simulink model "ACCSampleSimulink"  (R2022a)
settings: Solver=ode1  StartTime=0.0  StopTime=inf  FixedStep=0.001  RelTol=1e-3
model workspace (MAT data in the model file):
  ParaDataStoreNum = Simulink.Parameter
  ParaDataStoreNum.DataType = 'int32'
  ParaDataStoreNum.Complexity = 'real'
  ParaDataStoreNum.Dimensions = [0 0]
undefined symbols (not defined in the file): azimuth_angle, DataStoreNumPara, elevation_angle, GroundTruth_Objects, heading, id, range_bbox, range_center, shape, time, type, velocity, width
(part 1 of 2)
Description:
  | 22222
settings Model: Creator=15751  LastModifiedBy=jwd
settings SolverCC: AlgebraicLoopSolver=TrustRegion
settings OptimizationCC: LifeSpan=inf
settings DebuggingCC: MultiTaskRateTransMsg=warning  UnconnectedInputMsg=warning  UnconnectedOutputMsg=warning  UnconnectedLineMsg=warning  SFExecutionAtInitializationDiag=none  SFMachineParentedDataDiag=warning  ArithmeticOperatorsInVariantConditions=warning
settings SFSimCC: CustomCodeUndefinedFunction=UseInterfaceOnly
settings CodeAppCC: StateflowObjectComments=on

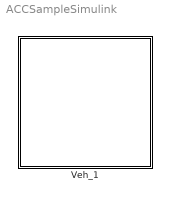
== system ACCSampleSimulink ==
  Veh_1 : Subsystem  Tag=PanoSim_System
      mask Display: image(imread('Sedan_2.jpg'));color('white');text(0,0,'Veh_1','HorizontalAlignment','left','verticalAlignment','bottom');color('red');text(0.1,0.1,'P','HorizontalAlignment','right','verticalAlignment','top');

== system ACCSampleSimulink/Veh_1 ==
  Algorithm : Subsystem
  AlgorithmControl : Subsystem
  ComplexVehicleModel : Subsystem
  Data Store Memory1 : DataStoreMemory  DataStoreName=DataStore_EGO_ALL  ReadBeforeWriteMsg=warning  WriteAfterWriteMsg=warning  WriteAfterReadMsg=warning  InitialValue=zeros(295,1)  ShowAdditionalParam=off  Dimensions=295
      settings: LockScale=on
  Data Store Memory2 : DataStoreMemory  DataStoreName=DataStore_COCKPIT_CONTROL  ReadBeforeWriteMsg=warning  WriteAfterWriteMsg=warning  WriteAfterReadMsg=warning  InitialValue=[0,0,0,0,0,0]  ShowAdditionalParam=off  Dimensions=6
      settings: LockScale=on
  Data Store Memory : DataStoreMemory  DataStoreName=DataStore_Ego_Control  ReadBeforeWriteMsg=warning  WriteAfterWriteMsg=warning  WriteAfterReadMsg=warning  InitialValue=[0,0,0,0,0,0]  ShowAdditionalParam=off  Dimensions=6
      settings: LockScale=on
  DriverModel : Subsystem  Tag=PanoSim_System
      mask Display: image(imread('driver.jpg'))
  GlobalVariable : Subsystem
  Sensors : Subsystem
  VehicleDataBus : Subsystem
  wires:
  Algorithm/3(LogDataOutput) -> VehicleDataBus/4(LogDataInput)
  Algorithm/2(GlobalVariableOutput) -> VehicleDataBus/2(GlobalVariable)
  Algorithm/1(ControlOutput) -> ComplexVehicleModel/1(Control)
  AlgorithmControl/1(AlgorithmControlOut) -> Algorithm/5(AlgorithmControlInput)
  GlobalVariable/1(Value) -> Algorithm/4(GlobalVariableInput)
  Sensors/1(SensorsOut) -> Algorithm/3(SensorsInput)
  DriverModel/1(DriverOut) -> Algorithm/2(ControlInput)
  [VehicleDynOut] -> Algorithm/1(VehDynInput)
  ComplexVehicleModel/1(Vehicle_Out) -> [VehicleDynOut], VehicleDataBus/1(VehicleDynOut)
  GlobalVariable/2(Original) -> VehicleDataBus/3(GlobalVariableOriginal)
  [VehicleDynOut] -> DriverModel/1(In1)

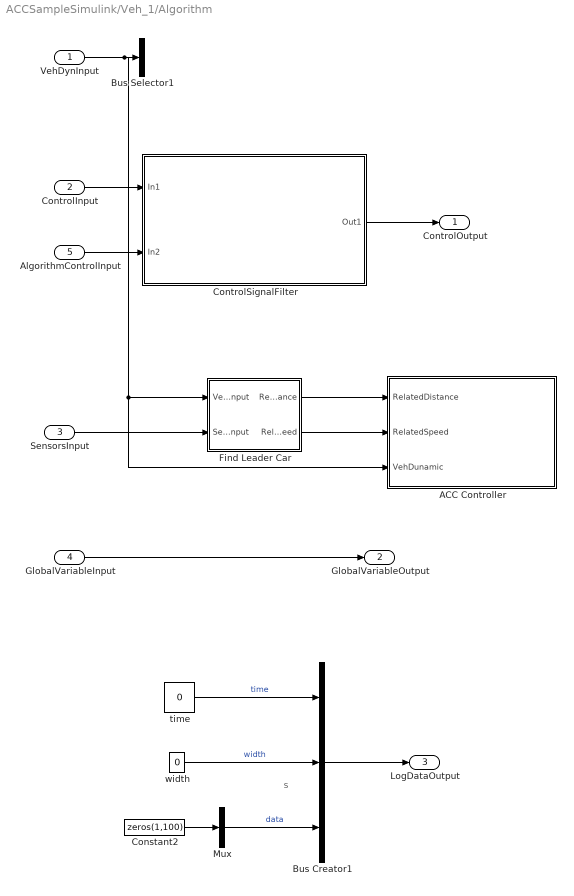
== system ACCSampleSimulink/Veh_1/Algorithm ==
  note: s
  VehDynInput : Inport
  ControlInput : Inport  Port=2
  SensorsInput : Inport  Port=3
  GlobalVariableInput : Inport  Port=4
  AlgorithmControlInput : Inport  Port=5
  " Find Leader Car" : Subsystem
  ACC Controller : Subsystem
  Bus Creator1 : BusCreator  Inputs=3
  Bus Selector1 : BusSelector  OutputSignals=ego
  Constant2 : Constant  Value=zeros(1,100)
  ControlSignalFilter : Subsystem
  Mux : Mux  Inputs=[100,]
  time : Constant  Value=0
  width : Constant  Value=0
  ControlOutput : Outport  VectorParamsAs1DForOutWhenUnconnected=off
  GlobalVariableOutput : Outport  Port=2  VectorParamsAs1DForOutWhenUnconnected=off
  LogDataOutput : Outport  Port=3  VectorParamsAs1DForOutWhenUnconnected=off
  wires:
  VehDynInput/1 -> ACC Controller/3(VehDunamic), " Find Leader Car"/1(VehDynInput), Bus Selector1/1
  ControlInput/1 -> ControlSignalFilter/1(In1)
  ControlSignalFilter/1(Out1) -> ControlOutput/1
  GlobalVariableInput/1 -> GlobalVariableOutput/1
  time/1 -> Bus Creator1/1  "time"
  Bus Creator1/1 -> LogDataOutput/1
  Constant2/1 -> Mux/1
  Mux/1 -> Bus Creator1/3  "data"
  width/1 -> Bus Creator1/2  "width"
  AlgorithmControlInput/1 -> ControlSignalFilter/2(In2)
  SensorsInput/1 -> " Find Leader Car"/2(SensorsInput)
  " Find Leader Car"/1(RelatedDistance) -> ACC Controller/1(RelatedDistance)
  " Find Leader Car"/2(RelatedSpeed) -> ACC Controller/2(RelatedSpeed)

== system ACCSampleSimulink/Veh_1/AlgorithmControl ==
  Bus{,2..5} (5 alike) : BusCreator  Inputs=3
  Bus1 : BusCreator  Inputs=5
  brake : S-Function  FunctionName=BusReader  Parameters='ego_control.brake','time@i,valid@b,brake@d','0.001','0.0'  SFunctionDeploymentMode=off  EnableBusSupport=off
  gear : S-Function  FunctionName=BusReader  Parameters='ego_control.gear','time@i,valid@b,gear@i','0.001','0.0'  SFunctionDeploymentMode=off  EnableBusSupport=off
  mode : S-Function  FunctionName=BusReader  Parameters='ego_control.mode','time@i,valid@b,mode@i','0.001','0.0'  SFunctionDeploymentMode=off  EnableBusSupport=off
  steer : S-Function  FunctionName=BusReader  Parameters='ego_control.steer','time@i,valid@b,steer@d','0.001','0.0'  SFunctionDeploymentMode=off  EnableBusSupport=off
  throttle : S-Function  FunctionName=BusReader  Parameters='ego_control.throttle','time@i,valid@b,throttle@d','0.001','0.0'  SFunctionDeploymentMode=off  EnableBusSupport=off
  AlgorithmControlOut : Outport  VectorParamsAs1DForOutWhenUnconnected=off
  wires:
  Bus1/1 -> AlgorithmControlOut/1
  Bus5/1 -> Bus1/1  "throttle"
  Bus4/1 -> Bus1/5  "gear"
  Bus3/1 -> Bus1/4  "mode"
  Bus2/1 -> Bus1/3  "steer"
  Bus/1 -> Bus1/2  "brake"
  gear/3 -> Bus4/3  "value"
  gear/2 -> Bus4/2  "valid"
  gear/1 -> Bus4/1  "time"
  mode/3 -> Bus3/3  "value"
  mode/2 -> Bus3/2  "valid"
  mode/1 -> Bus3/1  "time"
  steer/1 -> Bus2/1  "time"
  brake/1 -> Bus/1  "time"
  throttle/1 -> Bus5/1  "time"
  throttle/3 -> Bus5/3  "value"
  brake/3 -> Bus/3  "value"
  steer/3 -> Bus2/3  "value"
  throttle/2 -> Bus5/2  "valid"
  brake/2 -> Bus/2  "valid"
  steer/2 -> Bus2/2  "valid"

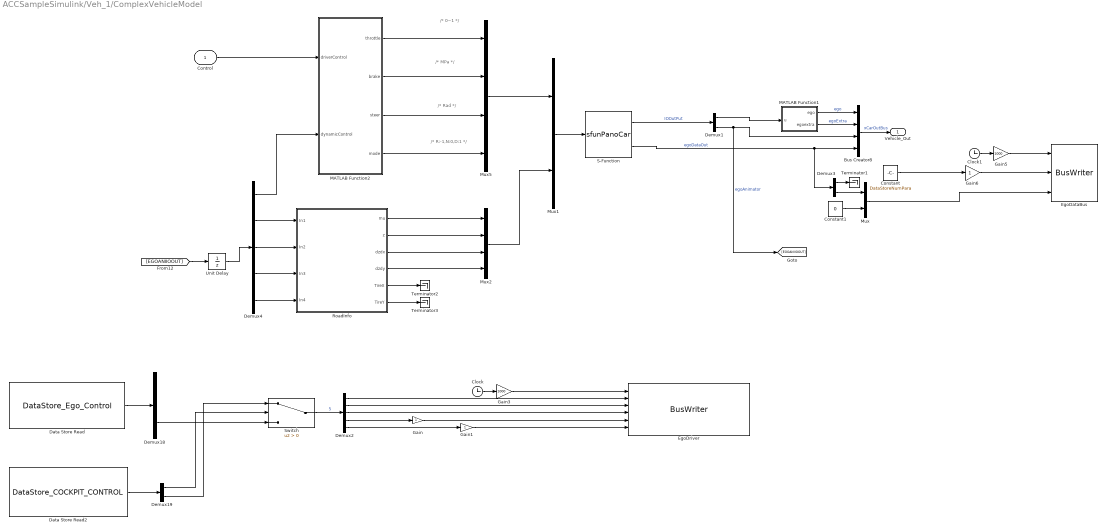
== system ACCSampleSimulink/Veh_1/ComplexVehicleModel ==
  note: /* MPa */
  note: /* 0~1 */
  note: /* R:-1,N:0,D:1 */
  note: /* Rad */
  Control : Inport
  Bus Creator8 : BusCreator  Inputs=4
  Clock : Clock
  Clock1 : Clock
  Constant : Constant  Value=DataStoreNumPara  VectorParams1D=off  OutDataTypeStr=double
  Constant1 : Constant  Value=0
  Data Store Read : DataStoreRead  DataStoreName=DataStore_Ego_Control  IndexOptions=Index vector (dialog)  Indices=1  OutputSizes=1
  Data Store Read2 : DataStoreRead  DataStoreName=DataStore_COCKPIT_CONTROL  IndexOptions=Index vector (dialog)  Indices=1  OutputSizes=1
  Demux1 : Demux  Outputs=[19,57]
  Demux18 : Demux  Outputs=[1,5]
  Demux19 : Demux  Outputs=[1,5]
  Demux2 : Demux  Outputs=5
  Demux3 : Demux  Outputs=[1,499]
  Demux4 : Demux  Outputs=[5,13,13,13,13]
  EgoDataBus : S-Function  FunctionName=BusWriter  Parameters='ego_data','time@i,500@[,data@d','0.01','0.0'  SFunctionDeploymentMode=off  EnableBusSupport=off
  EgoDriver : S-Function  FunctionName=BusWriter  Parameters='ego_driver','time@i,throttle@d,brake@d,steer@d,mode@i,gear@i','0.01','0.0'  SFunctionDeploymentMode=off  EnableBusSupport=off
  Gain : Gain  OutDataTypeStr=int32
  Gain1 : Gain  OutDataTypeStr=int32
  Gain3 : Gain  Gain=1000  OutDataTypeStr=Inherit: Inherit via back propagation  RndMeth=Nearest
  Gain5 : Gain  Gain=1000  OutDataTypeStr=Inherit: Inherit via back propagation  RndMeth=Nearest
  Gain6 : Gain  OutDataTypeStr=int32
  MATLAB Function1 : MATLAB Function  TreatAsAtomicUnit=on
  MATLAB Function2 : MATLAB Function  TreatAsAtomicUnit=on
  Mux : Mux  Inputs=[499,1]
  Mux1 : Mux  Inputs=[4,16]
  Mux2 : Mux
  Mux5 : Mux
  RoadInfo : Subsystem
  S-Function : S-Function  FunctionName=sfunPanoCar  SFunctionDeploymentMode=off  EnableBusSupport=off
  Switch : Switch  Criteria=u2 > Threshold  SaturateOnIntegerOverflow=off  InputSameDT=off
  Terminator1 : Terminator
  Terminator2 : Terminator
  Terminator3 : Terminator
  Unit Delay : UnitDelay  SampleTime=-1  HasFrameUpgradeWarning=on
  Vehicle_Out : Outport
  wires:
  MATLAB Function2/4(mode) -> Mux5/4
  MATLAB Function2/3(steer) -> Mux5/3
  MATLAB Function2/2(brake) -> Mux5/2
  MATLAB Function2/1(throttle) -> Mux5/1
  Demux4/4 -> RoadInfo/3(In3)
  Demux4/1 -> MATLAB Function2/2(dynamicControl)
  Demux4/2 -> RoadInfo/1(In1)
  Demux4/5 -> RoadInfo/4(In4)
  Unit Delay/1 -> Demux4/1
  Demux4/3 -> RoadInfo/2(In2)
  Mux/1 -> EgoDataBus/3
  Constant1/1 -> Mux/2
  Demux3/2 -> Mux/1
  Demux3/1 -> Terminator1/1
  Constant/1 -> Gain6/1
  Gain5/1 -> EgoDataBus/1
  Clock1/1 -> Gain5/1
  Gain6/1 -> EgoDataBus/2
  Demux19/2 -> Switch/1
  Data Store Read2/1 -> Demux19/1
  Data Store Read/1 -> Demux18/1
  Demux19/1 -> Switch/2
  Demux18/2 -> Switch/3
  Switch/1 -> Demux2/1  "5"
  Demux1/2 -> Bus Creator8/3, [EGOANIIOOUT]  "egoAnimator"
  MATLAB Function1/1(ego) -> Bus Creator8/1  "ego"
  Demux1/1 -> MATLAB Function1/1(u)
  MATLAB Function1/2(egoextra) -> Bus Creator8/2  "egoExtra"
  RoadInfo/6(TireY) -> Terminator3/1
  RoadInfo/5(TireX) -> Terminator2/1
  S-Function/2 -> Bus Creator8/4, Demux3/1  "egoDataOut"
  Gain1/1 -> EgoDriver/6
  Gain/1 -> EgoDriver/5
  Demux2/4 -> Gain/1
  Demux2/2 -> EgoDriver/3
  Control/1 -> MATLAB Function2/1(driverControl)
  Demux2/1 -> EgoDriver/2
  Demux2/3 -> EgoDriver/4
  Demux2/5 -> Gain1/1
  Gain3/1 -> EgoDriver/1
  Mux1/1 -> S-Function/1
  S-Function/1 -> Demux1/1  "IOOutPut"
  Bus Creator8/1 -> Vehicle_Out/1  "xCarOutBus"
  Mux5/1 -> Mux1/1
  Clock/1 -> Gain3/1
  Mux2/1 -> Mux1/2
  RoadInfo/3(dzdx) -> Mux2/3
  RoadInfo/1(mu) -> Mux2/1
  RoadInfo/2(z) -> Mux2/2
  RoadInfo/4(dzdy) -> Mux2/4
  [EGOANIIOOUT] -> Unit Delay/1

== system ACCSampleSimulink/Veh_1/DriverModel ==
  In1 : Inport
  DriverFilter : Subsystem
  DriverOut : Outport  VectorParamsAs1DForOutWhenUnconnected=off
  wires:
  DriverFilter/1(DriverOut) -> DriverOut/1

== system ACCSampleSimulink/Veh_1/GlobalVariable ==
  Bus : BusCreator  Inputs=2
  Variable : Subsystem
  Value : Outport  VectorParamsAs1DForOutWhenUnconnected=off
  Original : Outport  Port=2  VectorParamsAs1DForOutWhenUnconnected=off
  wires:
  Bus/1 -> Original/1
  Variable/2(Out2) -> Bus/2  "Time"
  Variable/1(Out1) -> Value/1, Bus/1  "Value"

== system ACCSampleSimulink/Veh_1/Sensors ==
  GroundTruth_Objects.0 : Subsystem
  SensorsBusCreator : BusCreator  Inputs=GroundTruth_Objects.0,
  sensor_template : Subsystem  Commented=on
  SensorsOut : Outport  VectorParamsAs1DForOutWhenUnconnected=off
  wires:
  SensorsBusCreator/1 -> SensorsOut/1
  GroundTruth_Objects.0/1(SensorOut) -> SensorsBusCreator/1  "GroundTruth_Objects.0"

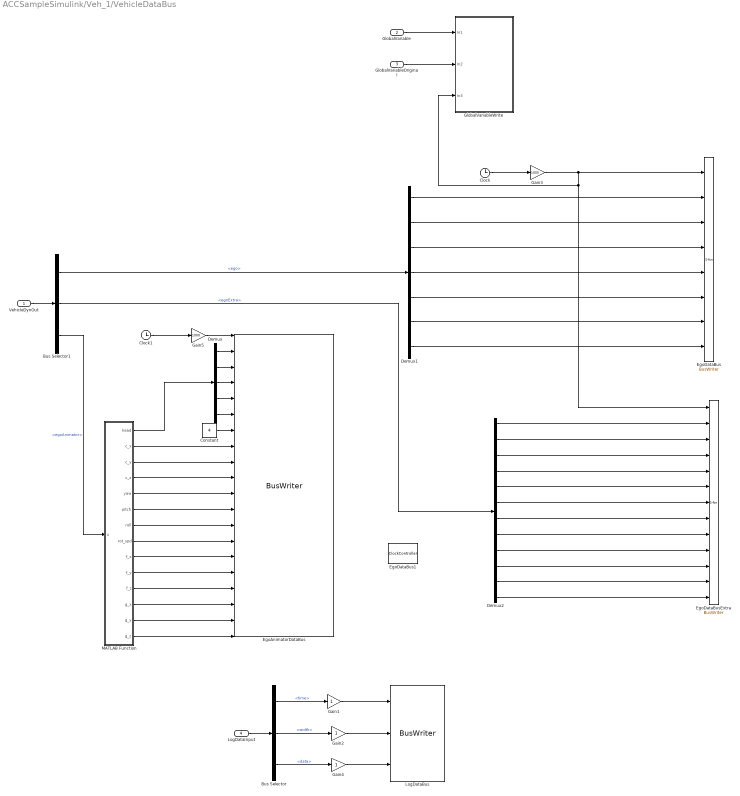
== system ACCSampleSimulink/Veh_1/VehicleDataBus ==
  VehicleDynOut : Inport
  GlobalVariable : Inport  Port=2
  GlobalVariableOriginal : Inport  Port=3
  LogDataInput : Inport  Port=4
  Bus Selector : BusSelector  OutputSignals=time,width,data
  Bus Selector1 : BusSelector  OutputSignals=ego,egoExtra,egoAnimator
  Clock : Clock
  Clock1 : Clock
  Constant : Constant  Value=4  OutDataTypeStr=int32
  Demux : Demux  Outputs=5
  Demux1 : Demux  Outputs=7
  Demux2 : Demux  Outputs=12
  EgoAnimatorDataBus : S-Function  FunctionName=BusWriter  Parameters='ego_animator','time@i,rot_spd@d,trans_gear@d,throttle@d,master@d,str@d,4@[,center_x@d,center_y@d,center_z@d,yaw@d,pitch@d,roll@d,rotation_spd@d,force_tire_x@d,force_tire_y@d,force_tire_z@d,gnd_x@d,gnd_y@d,gnd_z@d','0.01','0.0'  SFunctionDeploymentMode=off  EnableBusSupport=off
  EgoDataBus : S-Function  FunctionName=BusWriter  Parameters='ego','time@i,x@d,y@d,z@d,yaw@d,pitch@d,roll@d,speed@d','0.01','0.0'  SFunctionDeploymentMode=off  EnableBusSupport=off
  EgoDataBus1 : S-Function  FunctionName=ClockController  Parameters='step','0.01','0.0'  SFunctionDeploymentMode=off  EnableBusSupport=off
  EgoDataBusExtra : S-Function  FunctionName=BusWriter  Parameters='ego_extra','time@i,VX@d,VY@d,VZ@d,AVx@d,AVy@d,AVz@d,Ax@d,Ay@d,Az@d,AAx@d,AAy@d,AAz@d','0.01','0.0'  SFunctionDeploymentMode=off  EnableBusSupport=off
  Gain1 : Gain  OutDataTypeStr=int32  RndMeth=Nearest
  Gain2 : Gain  OutDataTypeStr=int32  RndMeth=Nearest
  Gain3 : Gain  Gain=1000  OutDataTypeStr=Inherit: Inherit via back propagation  RndMeth=Nearest
  Gain4 : Gain  OutDataTypeStr=double  RndMeth=Nearest
  Gain5 : Gain  Gain=1000  OutDataTypeStr=Inherit: Inherit via back propagation  RndMeth=Nearest
  GlobalVariableWrite : Subsystem
  LogDataBus : S-Function  FunctionName=BusWriter  Parameters='data','time@i,100@[,data@d','0.01','0.0'  SFunctionDeploymentMode=off  EnableBusSupport=off
  MATLAB Function : MATLAB Function  TreatAsAtomicUnit=on
  wires:
  Demux/5 -> EgoAnimatorDataBus/6
  MATLAB Function/14(g_z) -> EgoAnimatorDataBus/20
  MATLAB Function/13(g_y) -> EgoAnimatorDataBus/19
  MATLAB Function/12(g_x) -> EgoAnimatorDataBus/18
  MATLAB Function/11(f_z) -> EgoAnimatorDataBus/17
  MATLAB Function/10(f_y) -> EgoAnimatorDataBus/16
  MATLAB Function/9(f_x) -> EgoAnimatorDataBus/15
  MATLAB Function/8(rot_spd) -> EgoAnimatorDataBus/14
  MATLAB Function/7(roll) -> EgoAnimatorDataBus/13
  MATLAB Function/6(pitch) -> EgoAnimatorDataBus/12
  MATLAB Function/5(yaw) -> EgoAnimatorDataBus/11
  MATLAB Function/4(c_z) -> EgoAnimatorDataBus/10
  MATLAB Function/3(c_y) -> EgoAnimatorDataBus/9
  MATLAB Function/2(c_x) -> EgoAnimatorDataBus/8
  Constant/1 -> EgoAnimatorDataBus/7
  Demux/4 -> EgoAnimatorDataBus/5
  Demux/3 -> EgoAnimatorDataBus/4
  Demux/2 -> EgoAnimatorDataBus/3
  Demux/1 -> EgoAnimatorDataBus/2
  MATLAB Function/1(head) -> Demux/1
  Gain5/1 -> EgoAnimatorDataBus/1
  Clock1/1 -> Gain5/1
  Bus Selector1/3 -> MATLAB Function/1(u)  "<egoAnimator>"
  Bus Selector1/2 -> Demux2/1  "<egoExtra>"
  Bus Selector1/1 -> Demux1/1  "<ego>"
  Gain2/1 -> LogDataBus/2
  Bus Selector/2 -> Gain2/1  "<width>"
  Gain4/1 -> LogDataBus/3
  Bus Selector/1 -> Gain1/1  "<time>"
  Bus Selector/3 -> Gain4/1  "<data>"
  Gain1/1 -> LogDataBus/1
  LogDataInput/1 -> Bus Selector/1
  GlobalVariableOriginal/1 -> GlobalVariableWrite/2(In2)
  Gain3/1 -> EgoDataBus/1, EgoDataBusExtra/1, GlobalVariableWrite/3(In3)
  GlobalVariable/1 -> GlobalVariableWrite/1(In1)
  Demux2/12 -> EgoDataBusExtra/13
  Demux2/11 -> EgoDataBusExtra/12
  Demux2/10 -> EgoDataBusExtra/11
  Demux2/9 -> EgoDataBusExtra/10
  Demux2/8 -> EgoDataBusExtra/9
  Demux2/7 -> EgoDataBusExtra/8
  Demux2/6 -> EgoDataBusExtra/7
  Demux2/5 -> EgoDataBusExtra/6
  Demux2/4 -> EgoDataBusExtra/5
  Demux2/3 -> EgoDataBusExtra/4
  Demux2/2 -> EgoDataBusExtra/3
  Demux2/1 -> EgoDataBusExtra/2
  VehicleDynOut/1 -> Bus Selector1/1
  Clock/1 -> Gain3/1
  Demux1/1 -> EgoDataBus/2
  Demux1/2 -> EgoDataBus/3
  Demux1/3 -> EgoDataBus/4
  Demux1/4 -> EgoDataBus/5
  Demux1/5 -> EgoDataBus/6
  Demux1/6 -> EgoDataBus/7
  Demux1/7 -> EgoDataBus/8

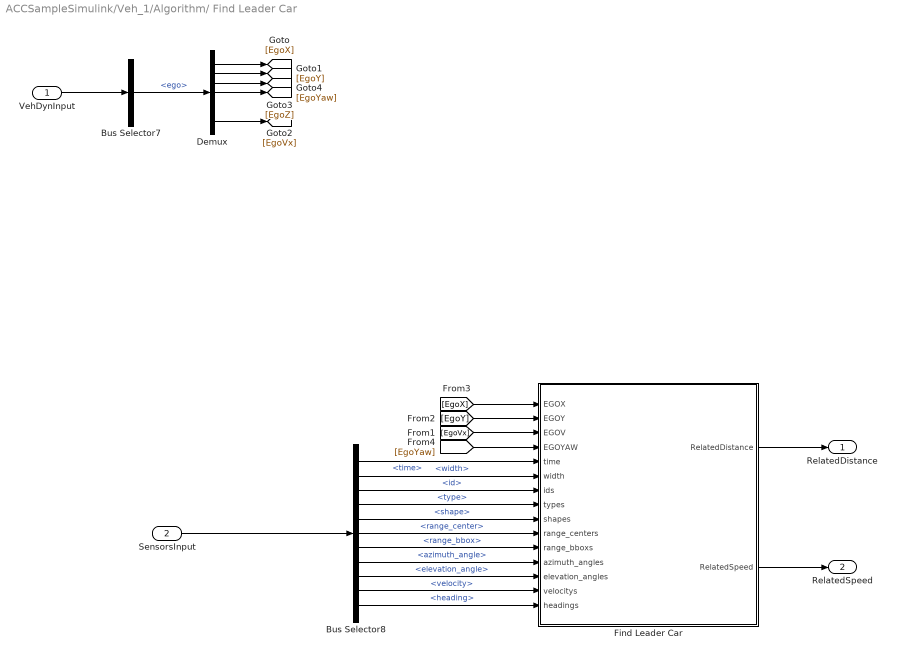
== system ACCSampleSimulink/Veh_1/Algorithm/ Find Leader Car ==
  VehDynInput : Inport
  SensorsInput : Inport  Port=2
  Bus Selector7 : BusSelector  OutputSignals=ego
  Bus Selector8 : BusSelector  OutputSignals=GroundTruth_Objects:0.time,GroundTruth_Objects:0.width,GroundTruth_Objects:0.id,GroundTruth_Objects:0.type,GroundTruth_Objects:0.shape,GroundTruth_Objects:0.range_center,GroundTruth_Objects:0.range_bbox,GroundTruth_Objects:0.azimuth_angle,GroundTruth_Objects:0.elevation_angle,GroundTruth_Objects:0.velocity,GroundTruth_Objects:0.heading
  Demux : Demux  Outputs=[1,1,1,1,1,1,1]
  Find Leader Car : MATLAB Function  TreatAsAtomicUnit=on
  RelatedDistance : Outport
  RelatedSpeed : Outport  Port=2
  wires:
  Find Leader Car/1(RelatedDistance) -> RelatedDistance/1
  Find Leader Car/2(RelatedSpeed) -> RelatedSpeed/1
  Bus Selector8/2 -> Find Leader Car/6(width)  "<width>"
  Bus Selector8/8 -> Find Leader Car/12(azimuth_angles)  "<azimuth_angle>"
  [EgoY] -> Find Leader Car/2(EGOY)
  Bus Selector8/1 -> Find Leader Car/5(time)  "<time>"
  [EgoX] -> Find Leader Car/1(EGOX)
  Bus Selector8/5 -> Find Leader Car/9(shapes)  "<shape>"
  Bus Selector8/4 -> Find Leader Car/8(types)  "<type>"
  Bus Selector8/3 -> Find Leader Car/7(ids)  "<id>"
  Bus Selector8/11 -> Find Leader Car/15(headings)  "<heading>"
  [EgoVx] -> Find Leader Car/3(EGOV)
  Bus Selector8/7 -> Find Leader Car/11(range_bboxs)  "<range_bbox>"
  [EgoYaw] -> Find Leader Car/4(EGOYAW)
  Bus Selector8/9 -> Find Leader Car/13(elevation_angles)  "<elevation_angle>"
  SensorsInput/1 -> Bus Selector8/1
  Bus Selector8/6 -> Find Leader Car/10(range_centers)  "<range_center>"
  Bus Selector8/10 -> Find Leader Car/14(velocitys)  "<velocity>"
  Demux/3 -> [EgoZ]
  Demux/1 -> [EgoX]
  Demux/7 -> [EgoVx]
  VehDynInput/1 -> Bus Selector7/1
  Demux/2 -> [EgoY]
  Demux/4 -> [EgoYaw]
  Bus Selector7/1 -> Demux/1  "<ego>"

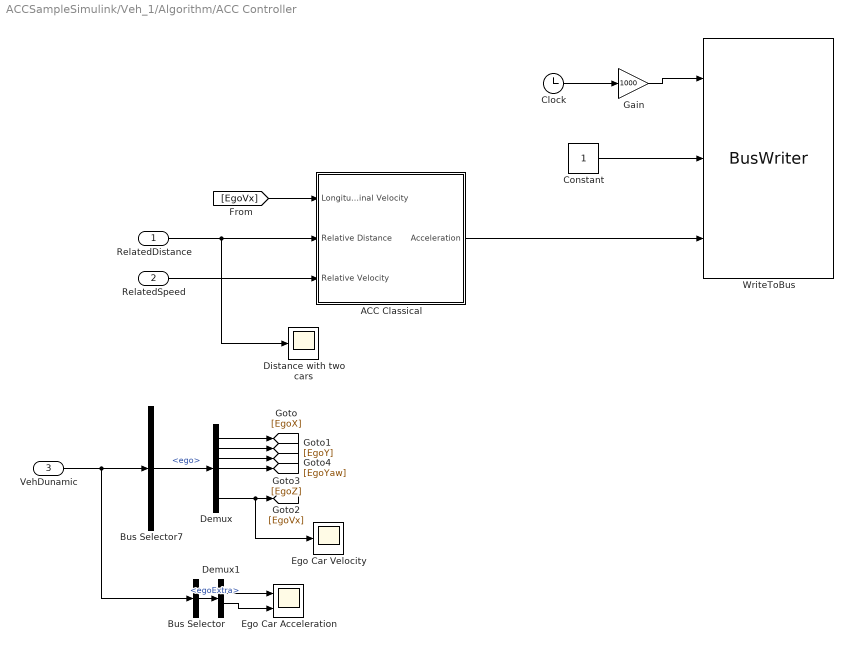
== system ACCSampleSimulink/Veh_1/Algorithm/ACC Controller ==
  RelatedDistance : Inport
  RelatedSpeed : Inport  Port=2
  VehDunamic : Inport  Port=3
  ACC Classical : Subsystem
  Bus Selector : BusSelector  OutputSignals=egoExtra
  Bus Selector7 : BusSelector  OutputSignals=ego
  Clock : Clock
  Constant : Constant  OutDataTypeStr=uint8
  Demux : Demux  Outputs=[1,1,1,1,1,1,1]
  Demux1 : Demux  Outputs=[6,1,1,4]
  Distance with two cars : Scope
  Ego Car Acceleration : Scope  NumInputPorts=2
  Ego Car Velocity : Scope
  Gain : Gain  Gain=1000  OutDataTypeStr=int32
  WriteToBus : S-Function  FunctionName=BusWriter  Parameters='xDriver_accel_input','time@i,valid@b,accel@d','0.01','0.0'  SFunctionDeploymentMode=off  EnableBusSupport=off
  wires:
  RelatedSpeed/1 -> ACC Classical/3("Relative Velocity ")
  RelatedDistance/1 -> Distance with two cars/1, ACC Classical/2(Relative Distance)
  Demux/1 -> [EgoX]
  Demux/4 -> [EgoYaw]
  Demux/2 -> [EgoY]
  VehDunamic/1 -> Bus Selector/1, Bus Selector7/1
  Demux/3 -> [EgoZ]
  [EgoVx] -> ACC Classical/1("Longitudinal Velocity ")
  Clock/1 -> Gain/1
  Gain/1 -> WriteToBus/1
  Constant/1 -> WriteToBus/2
  ACC Classical/1(" Acceleration") -> WriteToBus/3
  Bus Selector7/1 -> Demux/1  "<ego>"
  Demux1/3 -> Ego Car Acceleration/2
  Demux/7 -> Ego Car Velocity/1, [EgoVx]
  Bus Selector/1 -> Demux1/1  "<egoExtra>"
  Demux1/2 -> Ego Car Acceleration/1

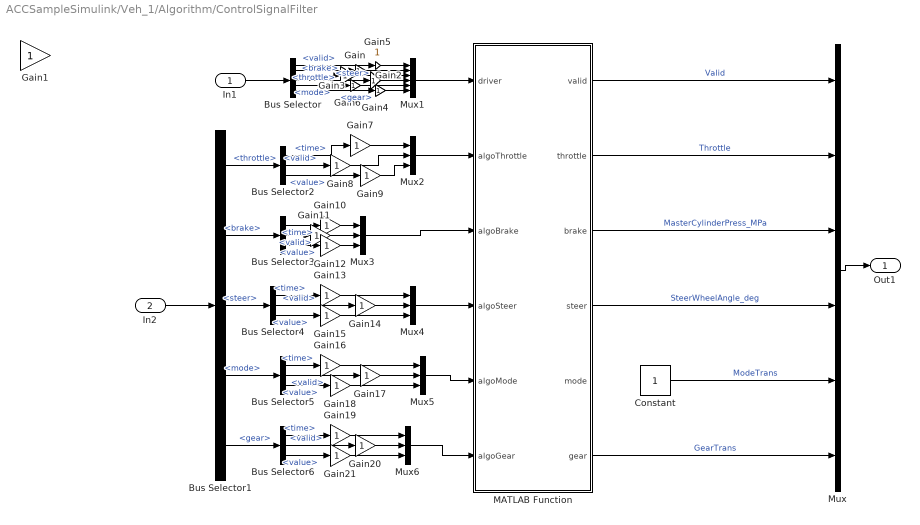
== system ACCSampleSimulink/Veh_1/Algorithm/ControlSignalFilter ==
  In1 : Inport
  In2 : Inport  Port=2
  Bus Selector : BusSelector  OutputSignals=valid,throttle,brake,steer,mode,gear
  Bus Selector1 : BusSelector  OutputSignals=throttle,brake,steer,mode,gear
  Bus Selector{2..6} (5 alike) : BusSelector  OutputSignals=time,valid,value
  Constant : Constant
  Gain{,2..21} (21 alike) : Gain  OutDataTypeStr=double
  Gain1 : Gain
  MATLAB Function : MATLAB Function  TreatAsAtomicUnit=on
  Mux : Mux  Inputs=6
  Mux1 : Mux  Inputs=6
  Mux{2..6} (5 alike) : Mux  Inputs=3
  Out1 : Outport  VectorParamsAs1DForOutWhenUnconnected=off
  wires:
  In1/1 -> Bus Selector/1
  Mux/1 -> Out1/1
  MATLAB Function/2(throttle) -> Mux/2  "Throttle"
  MATLAB Function/4(steer) -> Mux/4  "SteerWheelAngle_deg"
  MATLAB Function/1(valid) -> Mux/1  "Valid"
  Constant/1 -> Mux/5  "ModeTrans"
  MATLAB Function/6(gear) -> Mux/6  "GearTrans"
  In2/1 -> Bus Selector1/1
  Bus Selector1/1 -> Bus Selector2/1  "<throttle>"
  Bus Selector1/2 -> Bus Selector3/1  "<brake>"
  Bus Selector1/3 -> Bus Selector4/1  "<steer>"
  Bus Selector1/4 -> Bus Selector5/1  "<mode>"
  Bus Selector1/5 -> Bus Selector6/1  "<gear>"
  MATLAB Function/3(brake) -> Mux/3  "MasterCylinderPress_MPa"
  Bus Selector/1 -> Gain5/1  "<valid>"
  Bus Selector/2 -> Gain/1  "<throttle>"
  Bus Selector/3 -> Gain6/1  "<brake>"
  Bus Selector/4 -> Gain4/1  "<steer>"
  Bus Selector/5 -> Gain3/1  "<mode>"
  Bus Selector/6 -> Gain2/1  "<gear>"
  Mux1/1 -> MATLAB Function/1(driver)
  Bus Selector2/1 -> Gain7/1  "<time>"
  Bus Selector2/2 -> Gain8/1  "<valid>"
  Bus Selector2/3 -> Gain9/1  "<value>"
  Mux2/1 -> MATLAB Function/2(algoThrottle)
  Bus Selector3/1 -> Gain10/1  "<time>"
  Bus Selector3/2 -> Gain11/1  "<valid>"
  Bus Selector3/3 -> Gain12/1  "<value>"
  Mux3/1 -> MATLAB Function/3(algoBrake)
  Bus Selector4/1 -> Gain13/1  "<time>"
  Bus Selector4/2 -> Gain14/1  "<valid>"
  Bus Selector4/3 -> Gain15/1  "<value>"
  Mux4/1 -> MATLAB Function/4(algoSteer)
  Bus Selector5/1 -> Gain16/1  "<time>"
  Bus Selector5/2 -> Gain17/1  "<valid>"
  Bus Selector5/3 -> Gain18/1  "<value>"
  Mux5/1 -> MATLAB Function/5(algoMode)
  Bus Selector6/1 -> Gain19/1  "<time>"
  Bus Selector6/2 -> Gain20/1  "<valid>"
  Bus Selector6/3 -> Gain21/1  "<value>"
  Mux6/1 -> MATLAB Function/6(algoGear)
  Gain/1 -> Mux1/2
  Gain2/1 -> Mux1/6
  Gain3/1 -> Mux1/5
  Gain4/1 -> Mux1/4
  Gain5/1 -> Mux1/1
  Gain6/1 -> Mux1/3
  Gain7/1 -> Mux2/1
  Gain8/1 -> Mux2/2
  Gain9/1 -> Mux2/3
  Gain10/1 -> Mux3/1
  Gain11/1 -> Mux3/2
  Gain12/1 -> Mux3/3
  Gain13/1 -> Mux4/1
  Gain14/1 -> Mux4/2
  Gain15/1 -> Mux4/3
  Gain16/1 -> Mux5/1
  Gain17/1 -> Mux5/2
  Gain18/1 -> Mux5/3
  Gain19/1 -> Mux6/1
  Gain20/1 -> Mux6/2
  Gain21/1 -> Mux6/3

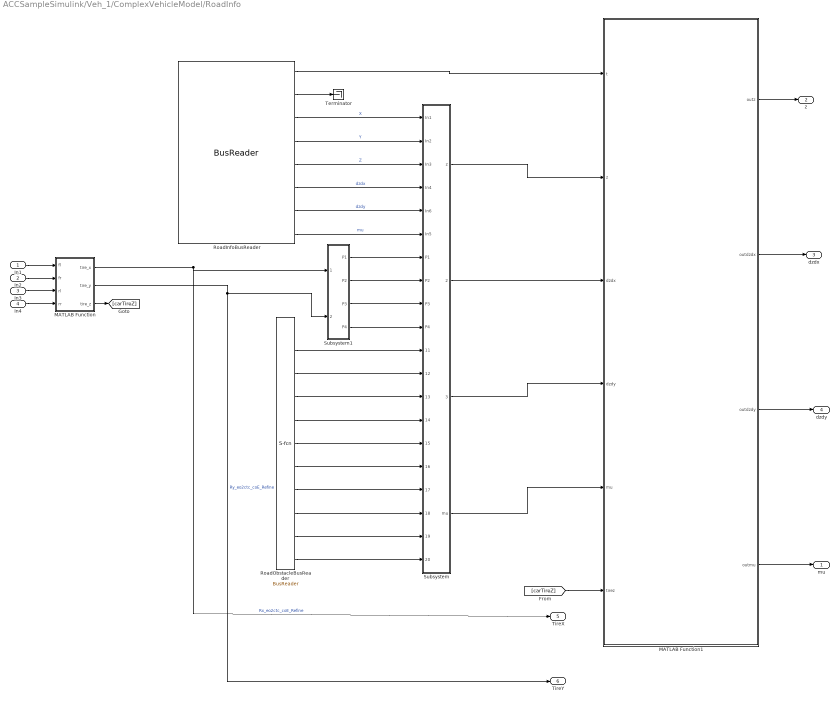
== system ACCSampleSimulink/Veh_1/ComplexVehicleModel/RoadInfo ==
  In1 : Inport
  In2 : Inport  Port=2
  In3 : Inport  Port=3
  In4 : Inport  Port=4
  MATLAB Function : MATLAB Function  TreatAsAtomicUnit=on
  MATLAB Function1 : MATLAB Function  TreatAsAtomicUnit=on
  RoadInfoBusReader : S-Function  FunctionName=BusReader  Parameters='road_info','time@i,16@[,x@d,y@d,z@d,dzdx@d,dzdy@d,mu@d','0.001','0.0'  SFunctionDeploymentMode=off  EnableBusSupport=off
  RoadObstacleBusReader : S-Function  FunctionName=BusReader  Parameters='road_obstacle','time@i,4@[,x1@d,y1@d,x2@d,y2@d,x3@d,y3@d,x4@d,y4@d,z@d','0.001','0.0'  SFunctionDeploymentMode=off  EnableBusSupport=off
  Subsystem : Subsystem
  Subsystem1 : Subsystem
  Terminator : Terminator
  mu : Outport  VectorParamsAs1DForOutWhenUnconnected=off
  z : Outport  Port=2  VectorParamsAs1DForOutWhenUnconnected=off
  dzdx : Outport  Port=3  VectorParamsAs1DForOutWhenUnconnected=off
  dzdy : Outport  Port=4  VectorParamsAs1DForOutWhenUnconnected=off
  TireX : Outport  Port=5  VectorParamsAs1DForOutWhenUnconnected=off
  TireY : Outport  Port=6  VectorParamsAs1DForOutWhenUnconnected=off
  wires:
  In1/1 -> MATLAB Function/1(fl)
  In2/1 -> MATLAB Function/2(fr)
  In3/1 -> MATLAB Function/3(rl)
  In4/1 -> MATLAB Function/4(rr)
  MATLAB Function1/4(outmu) -> mu/1
  MATLAB Function1/3(outdzdy) -> dzdy/1
  MATLAB Function1/2(outdzdx) -> dzdx/1
  MATLAB Function1/1(outz) -> z/1
  [carTireZ] -> MATLAB Function1/6(tirez)
  RoadInfoBusReader/1 -> MATLAB Function1/1(t)
  RoadInfoBusReader/2 -> Terminator/1
  MATLAB Function/3(tire_z) -> [carTireZ]
  RoadObstacleBusReader/11 -> Subsystem/20(In20)
  RoadObstacleBusReader/10 -> Subsystem/19(In19)
  RoadObstacleBusReader/9 -> Subsystem/18(In18)
  RoadObstacleBusReader/8 -> Subsystem/17(In17)
  RoadObstacleBusReader/7 -> Subsystem/16(In16)
  RoadObstacleBusReader/6 -> Subsystem/15(In15)
  RoadObstacleBusReader/5 -> Subsystem/14(In14)
  RoadObstacleBusReader/4 -> Subsystem/13(In13)
  RoadObstacleBusReader/3 -> Subsystem/12(In12)
  RoadObstacleBusReader/2 -> Subsystem/11(In11)
  RoadInfoBusReader/3 -> Subsystem/1(In1)  "X"
  RoadInfoBusReader/4 -> Subsystem/2(In2)  "Y"
  RoadInfoBusReader/5 -> Subsystem/3(In3)  "Z"
  RoadInfoBusReader/6 -> Subsystem/4(In4)  "dzdx"
  RoadInfoBusReader/7 -> Subsystem/5(In6)  "dzdy"
  RoadInfoBusReader/8 -> Subsystem/6(In5)  "mu"
  Subsystem/4(mu) -> MATLAB Function1/5(mu)
  Subsystem/3(dzdy) -> MATLAB Function1/4(dzdy)
  Subsystem/1(z) -> MATLAB Function1/2(z)
  Subsystem/2(dzdx) -> MATLAB Function1/3(dzdx)
  MATLAB Function/2(tire_y) -> Subsystem1/2(Ry_eo2ctc_coE_Refine), TireY/1  "Ry_eo2ctc_coE_Refine"
  MATLAB Function/1(tire_x) -> Subsystem1/1(Rx_eo2ctc_coE_Refine), TireX/1  "Rx_eo2ctc_coE_Refine"
  Subsystem1/1(P1) -> Subsystem/7(P1)
  Subsystem1/2(P2) -> Subsystem/8(P2)
  Subsystem1/3(P3) -> Subsystem/9(P3)
  Subsystem1/4(P4) -> Subsystem/10(P4)

== system ACCSampleSimulink/Veh_1/DriverModel/DriverFilter ==
  note: DriverBusCreator
  Bus Creator2 : BusCreator  Inputs=6
  Bus Selector : BusSelector  OutputSignals=valid,throttle,brake,steer,mode,gear
  Data Store Write : DataStoreWrite  DataStoreName=DataStore_Ego_Control  IndexOptions=Index vector (dialog)  Indices=1  OutputSizes=1
  EgoControlBus : S-Function  FunctionName=BusReader  Parameters='ego_control','time@i,valid@b,throttle@d,brake@d,steer@d,mode@i,gear@i','0.001','0.0'  SFunctionDeploymentMode=off  EnableBusSupport=off
  Gain : Gain  OutDataTypeStr=double
  Gain1 : Gain  OutDataTypeStr=double
  Gain2 : Gain  OutDataTypeStr=double
  Mux : Mux  Inputs=6
  DriverOut : Outport  VectorParamsAs1DForOutWhenUnconnected=off
  wires:
  Bus Selector/6 -> Gain1/1  "<gear>"
  Bus Selector/1 -> Gain2/1  "<valid>"
  Bus Creator2/1 -> DriverOut/1, Bus Selector/1
  Gain/1 -> Mux/5
  Bus Selector/2 -> Mux/2  "<throttle>"
  Bus Selector/5 -> Gain/1  "<mode>"
  Gain1/1 -> Mux/6
  Gain2/1 -> Mux/1
  Bus Selector/4 -> Mux/4  "<steer>"
  Mux/1 -> Data Store Write/1
  Bus Selector/3 -> Mux/3  "<brake>"
  EgoControlBus/4 -> Bus Creator2/3  "brake"
  EgoControlBus/5 -> Bus Creator2/4  "steer"
  EgoControlBus/3 -> Bus Creator2/2  "throttle"
  EgoControlBus/2 -> Bus Creator2/1  "valid"
  EgoControlBus/6 -> Bus Creator2/5  "mode"
  EgoControlBus/7 -> Bus Creator2/6  "gear"

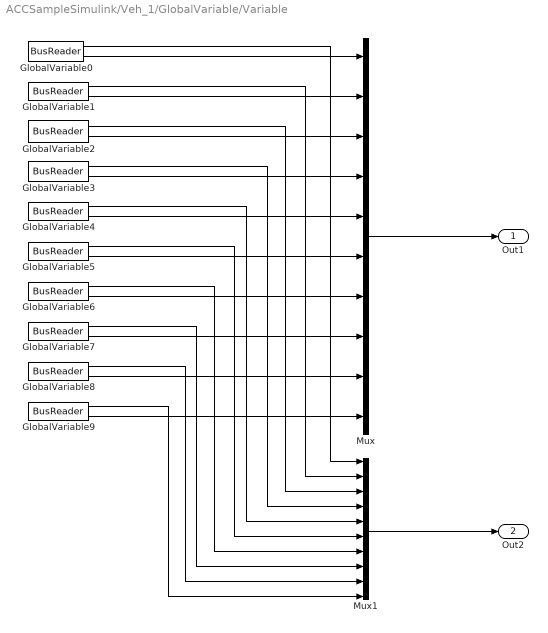
== system ACCSampleSimulink/Veh_1/GlobalVariable/Variable ==
  GlobalVariable0 : S-Function  FunctionName=BusReader  Parameters='global.0','time@i,variable@d','0.01','0.0'  SFunctionDeploymentMode=off  EnableBusSupport=off
  GlobalVariable1 : S-Function  FunctionName=BusReader  Parameters='global.1','time@i,variable@d','0.01','0.0'  SFunctionDeploymentMode=off  EnableBusSupport=off
  GlobalVariable2 : S-Function  FunctionName=BusReader  Parameters='global.2','time@i,variable@d','0.01','0.0'  SFunctionDeploymentMode=off  EnableBusSupport=off
  GlobalVariable3 : S-Function  FunctionName=BusReader  Parameters='global.3','time@i,variable@d','0.01','0.0'  SFunctionDeploymentMode=off  EnableBusSupport=off
  GlobalVariable4 : S-Function  FunctionName=BusReader  Parameters='global.4','time@i,variable@d','0.01','0.0'  SFunctionDeploymentMode=off  EnableBusSupport=off
  GlobalVariable5 : S-Function  FunctionName=BusReader  Parameters='global.5','time@i,variable@d','0.01','0.0'  SFunctionDeploymentMode=off  EnableBusSupport=off
  GlobalVariable6 : S-Function  FunctionName=BusReader  Parameters='global.6','time@i,variable@d','0.01','0.0'  SFunctionDeploymentMode=off  EnableBusSupport=off
  GlobalVariable7 : S-Function  FunctionName=BusReader  Parameters='global.7','time@i,variable@d','0.01','0.0'  SFunctionDeploymentMode=off  EnableBusSupport=off
  GlobalVariable8 : S-Function  FunctionName=BusReader  Parameters='global.8','time@i,variable@d','0.01','0.0'  SFunctionDeploymentMode=off  EnableBusSupport=off
  GlobalVariable9 : S-Function  FunctionName=BusReader  Parameters='global.9','time@i,variable@d','0.01','0.0'  SFunctionDeploymentMode=off  EnableBusSupport=off
  Mux : Mux  Inputs=10
  Mux1 : Mux  Inputs=10
  Out1 : Outport  VectorParamsAs1DForOutWhenUnconnected=off
  Out2 : Outport  Port=2  VectorParamsAs1DForOutWhenUnconnected=off
  wires:
  GlobalVariable9/1 -> Mux1/10
  GlobalVariable8/1 -> Mux1/9
  GlobalVariable7/1 -> Mux1/8
  GlobalVariable6/1 -> Mux1/7
  GlobalVariable5/1 -> Mux1/6
  GlobalVariable4/1 -> Mux1/5
  GlobalVariable3/1 -> Mux1/4
  GlobalVariable2/1 -> Mux1/3
  GlobalVariable1/1 -> Mux1/2
  GlobalVariable0/1 -> Mux1/1
  Mux1/1 -> Out2/1
  GlobalVariable9/2 -> Mux/10
  GlobalVariable8/2 -> Mux/9
  GlobalVariable7/2 -> Mux/8
  GlobalVariable6/2 -> Mux/7
  GlobalVariable5/2 -> Mux/6
  GlobalVariable4/2 -> Mux/5
  GlobalVariable3/2 -> Mux/4
  GlobalVariable2/2 -> Mux/3
  GlobalVariable1/2 -> Mux/2
  Mux/1 -> Out1/1
  GlobalVariable0/2 -> Mux/1

== system ACCSampleSimulink/Veh_1/Sensors/GroundTruth_Objects.0 ==
  BusCreator : BusCreator  Inputs=time,width,id,type,shape,range_center,range_bbox,azimuth_angle,elevation_angle,velocity,heading
  SensorBus : S-Function  FunctionName=BusReader  Parameters='GroundTruth_Objects.0','time@i,100@[,id@i,type@b,shape@i,range_center@f,range_bbox@f,azimuth_angle@f,elevation_angle@f,velocity@f,heading@f','0.01','0.0'  SFunctionDeploymentMode=off  EnableBusSupport=off
  SensorOut : Outport  VectorParamsAs1DForOutWhenUnconnected=off
  wires:
  SensorBus/11 -> BusCreator/11  "heading"
  SensorBus/10 -> BusCreator/10  "velocity"
  SensorBus/9 -> BusCreator/9  "elevation_angle"
  SensorBus/8 -> BusCreator/8  "azimuth_angle"
  SensorBus/7 -> BusCreator/7  "range_bbox"
  SensorBus/6 -> BusCreator/6  "range_center"
  SensorBus/5 -> BusCreator/5  "shape"
  SensorBus/4 -> BusCreator/4  "type"
  SensorBus/3 -> BusCreator/3  "id"
  SensorBus/2 -> BusCreator/2  "width"
  SensorBus/1 -> BusCreator/1  "time"
  BusCreator/1 -> SensorOut/1

== system ACCSampleSimulink/Veh_1/Sensors/sensor_template ==
  BusCreator : BusCreator  Inputs=8
  SensorBus : S-Function  FunctionName=BusReader  Parameters='mmwradar.0','time@i,64@[,angle@d,distance@d,speed@d,type@b,energy@d,id@i','0.1','0.0'  SFunctionDeploymentMode=off  EnableBusSupport=off
  SensorOut : Outport  VectorParamsAs1DForOutWhenUnconnected=off
  wires:
  BusCreator/1 -> SensorOut/1

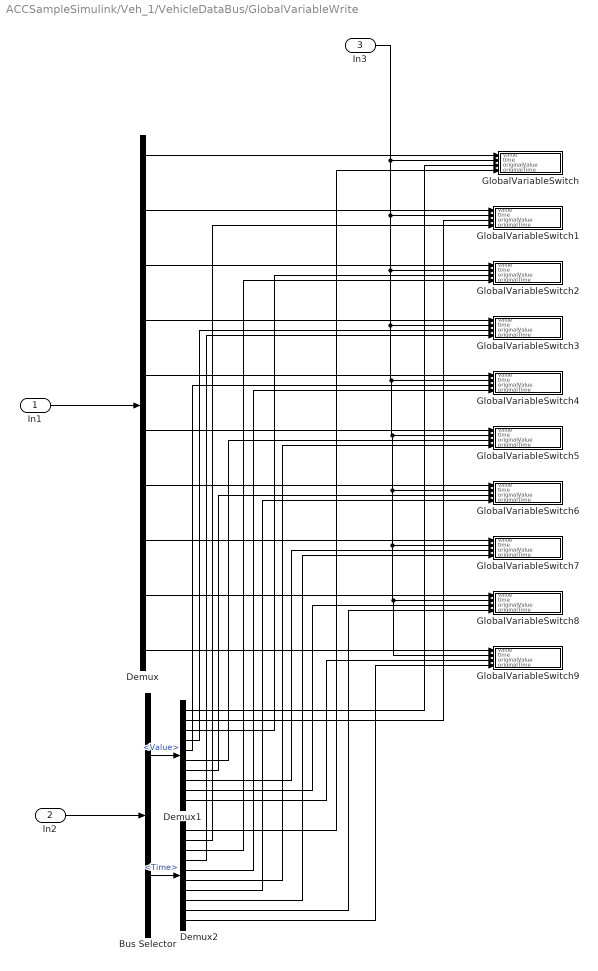
== system ACCSampleSimulink/Veh_1/VehicleDataBus/GlobalVariableWrite ==
  In1 : Inport
  In2 : Inport  Port=2
  In3 : Inport  Port=3
  Bus Selector : BusSelector  OutputSignals=Value,Time
  Demux : Demux  Outputs=10
  Demux1 : Demux  Outputs=10
  Demux2 : Demux  Outputs=10
  GlobalVariableSwitch : Subsystem
  GlobalVariableSwitch1 : Subsystem
  GlobalVariableSwitch2 : Subsystem
  GlobalVariableSwitch3 : Subsystem
  GlobalVariableSwitch4 : Subsystem
  GlobalVariableSwitch5 : Subsystem
  GlobalVariableSwitch6 : Subsystem
  GlobalVariableSwitch7 : Subsystem
  GlobalVariableSwitch8 : Subsystem
  GlobalVariableSwitch9 : Subsystem
  wires:
  Demux2/10 -> GlobalVariableSwitch9/4(originalTime)
  Demux1/10 -> GlobalVariableSwitch9/3(originalValue)
  Demux/10 -> GlobalVariableSwitch9/1(value)
  Demux2/9 -> GlobalVariableSwitch8/4(originalTime)
  Demux1/9 -> GlobalVariableSwitch8/3(originalValue)
  Demux/9 -> GlobalVariableSwitch8/1(value)
  Demux2/8 -> GlobalVariableSwitch7/4(originalTime)
  Demux1/8 -> GlobalVariableSwitch7/3(originalValue)
  Demux/8 -> GlobalVariableSwitch7/1(value)
  Demux2/7 -> GlobalVariableSwitch6/4(originalTime)
  Demux1/7 -> GlobalVariableSwitch6/3(originalValue)
  Demux/7 -> GlobalVariableSwitch6/1(value)
  Demux2/6 -> GlobalVariableSwitch5/4(originalTime)
  Demux1/6 -> GlobalVariableSwitch5/3(originalValue)
  Demux/6 -> GlobalVariableSwitch5/1(value)
  Demux2/5 -> GlobalVariableSwitch4/4(originalTime)
  Demux1/5 -> GlobalVariableSwitch4/3(originalValue)
  Demux/5 -> GlobalVariableSwitch4/1(value)
  Demux2/4 -> GlobalVariableSwitch3/4(originalTime)
  Demux1/4 -> GlobalVariableSwitch3/3(originalValue)
  Demux/4 -> GlobalVariableSwitch3/1(value)
  Demux2/3 -> GlobalVariableSwitch2/4(originalTime)
  Demux1/3 -> GlobalVariableSwitch2/3(originalValue)
  Demux/3 -> GlobalVariableSwitch2/1(value)
  Demux2/2 -> GlobalVariableSwitch1/4(originalTime)
  Demux1/2 -> GlobalVariableSwitch1/3(originalValue)
  Demux/2 -> GlobalVariableSwitch1/1(value)
  Demux2/1 -> GlobalVariableSwitch/4(originalTime)
  Demux1/1 -> GlobalVariableSwitch/3(originalValue)
  Demux/1 -> GlobalVariableSwitch/1(value)
  Bus Selector/2 -> Demux2/1  "<Time>"
  Bus Selector/1 -> Demux1/1  "<Value>"
  In2/1 -> Bus Selector/1
  In1/1 -> Demux/1
  In3/1 -> GlobalVariableSwitch/2(time), GlobalVariableSwitch1/2(time), GlobalVariableSwitch2/2(time), GlobalVariableSwitch3/2(time), GlobalVariableSwitch4/2(time), GlobalVariableSwitch5/2(time), GlobalVariableSwitch6/2(time), GlobalVariableSwitch7/2(time), GlobalVariableSwitch8/2(time), GlobalVariableSwitch9/2(time)

== system ACCSampleSimulink/Veh_1/Algorithm/ACC Controller/ACC Classical ==
  "Longitudinal Velocity " : Inport
  Relative Distance : Inport  Port=2
  "Relative Velocity " : Inport  Port=3
  ACC Classical : Subsystem  TreatAsAtomicUnit=on  VariantControl=controller_type == 1
      settings: RTWFileNameOpts=Use function name
  " Acceleration" : Outport  VectorParamsAs1DForOutWhenUnconnected=off
  wires:
  "Longitudinal Velocity "/1 -> ACC Classical/1(Longitudinal Velocity)
  Relative Distance/1 -> ACC Classical/2(Relative Distance)
  "Relative Velocity "/1 -> ACC Classical/3(Relative Velocity)
  ACC Classical/1(Acceleration) -> " Acceleration"/1

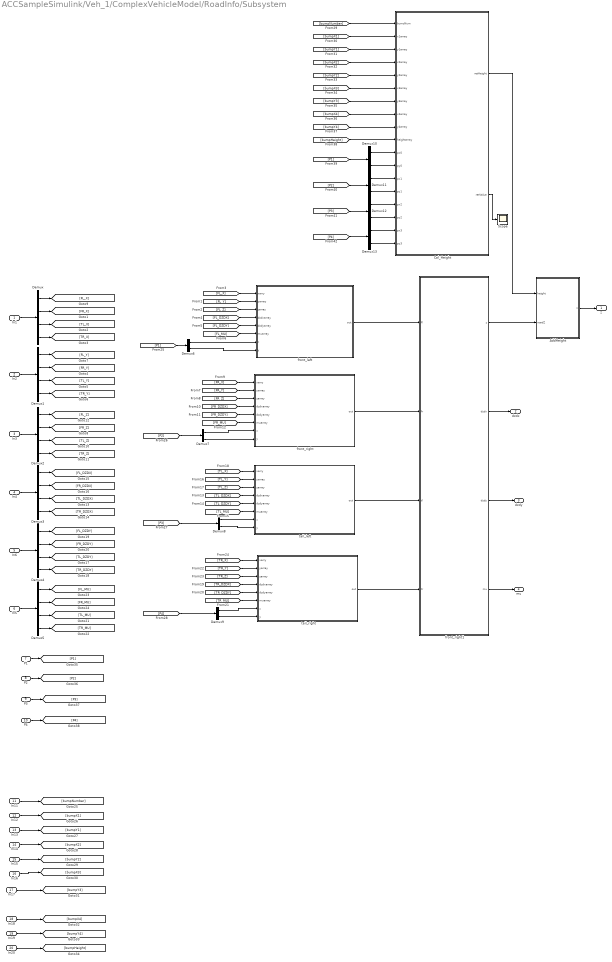
== system ACCSampleSimulink/Veh_1/ComplexVehicleModel/RoadInfo/Subsystem ==
  In1 : Inport
  In2 : Inport  Port=2
  In3 : Inport  Port=3
  In4 : Inport  Port=4
  In6 : Inport  Port=5
  In5 : Inport  Port=6
  P1 : Inport  Port=7
  P2 : Inport  Port=8
  P3 : Inport  Port=9
  P4 : Inport  Port=10
  In11 : Inport  Port=11
  In12 : Inport  Port=12
  In13 : Inport  Port=13
  In14 : Inport  Port=14
  In15 : Inport  Port=15
  In16 : Inport  Port=16
  In17 : Inport  Port=17
  In18 : Inport  Port=18
  In19 : Inport  Port=19
  In20 : Inport  Port=20
  AddHeight : MATLAB Function  TreatAsAtomicUnit=on
  Cal_Height : MATLAB Function  TreatAsAtomicUnit=on
  Demux{,1..5} (6 alike) : Demux
  Demux{6..13} (8 alike) : Demux  Outputs=2
  Scope : Scope
  front_left : MATLAB Function  TreatAsAtomicUnit=on
  front_right : MATLAB Function  TreatAsAtomicUnit=on
  front_right1 : MATLAB Function  TreatAsAtomicUnit=on
  tail_left : MATLAB Function  TreatAsAtomicUnit=on
  tail_right : MATLAB Function  TreatAsAtomicUnit=on
  z : Outport  VectorParamsAs1DForOutWhenUnconnected=off
  dzdx : Outport  Port=2  VectorParamsAs1DForOutWhenUnconnected=off
  dzdy : Outport  Port=3  VectorParamsAs1DForOutWhenUnconnected=off
  mu : Outport  Port=4  VectorParamsAs1DForOutWhenUnconnected=off
  wires:
  Cal_Height/2(retValue) -> Scope/1
  AddHeight/1(z) -> z/1
  Cal_Height/1(retHeight) -> AddHeight/1(height)
  [bumpY3] -> Cal_Height/7(y3array)
  Demux11/1 -> Cal_Height/13(px1)
  [bumpHeight] -> Cal_Height/10(heightarray)
  [bumpX1] -> Cal_Height/2(x1array)
  Demux11/2 -> Cal_Height/14(py1)
  [bumpY1] -> Cal_Height/3(y1array)
  [P2] -> Demux11/1
  Demux10/1 -> Cal_Height/11(px0)
  [bumpX3] -> Cal_Height/6(x3array)
  [P3] -> Demux12/1
  Demux10/2 -> Cal_Height/12(py0)
  [bumpNumber] -> Cal_Height/1(bumsNum)
  Demux12/1 -> Cal_Height/15(px2)
  [P4] -> Demux13/1
  Demux12/2 -> Cal_Height/16(py2)
  [bumpY4] -> Cal_Height/9(y4array)
  [bumpX4] -> Cal_Height/8(x4array)
  [P1] -> Demux10/1
  [bumpX2] -> Cal_Height/4(x2array)
  Demux13/1 -> Cal_Height/17(px3)
  Demux13/2 -> Cal_Height/18(py3)
  [bumpY2] -> Cal_Height/5(y2array)
  [P4] -> Demux9/1
  [P3] -> Demux8/1
  [P2] -> Demux7/1
  [P1] -> Demux6/1
  In20/1 -> [bumpHeight]
  In19/1 -> [bumpY4]
  In18/1 -> [bumpX4]
  In17/1 -> [bumpY3]
  In16/1 -> [bumpX3]
  In15/1 -> [bumpY2]
  In14/1 -> [bumpX2]
  In13/1 -> [bumpY1]
  In12/1 -> [bumpX1]
  In11/1 -> [bumpNumber]
  In1/1 -> Demux/1
  Demux/1 -> [FL_X]
  Demux/2 -> [FR_X]
  Demux/3 -> [TL_X]
  Demux/4 -> [TR_X]
  Demux1/1 -> [FL_Y]
  Demux1/3 -> [TL_Y]
  Demux1/4 -> [TR_Y]
  Demux1/2 -> [FR_Y]
  In2/1 -> Demux1/1
  In3/1 -> Demux2/1
  Demux2/4 -> [TR_Z]
  Demux2/3 -> [TL_Z]
  Demux2/2 -> [FR_Z]
  Demux2/1 -> [FL_Z]
  Demux3/4 -> [TR_DZDX]
  In4/1 -> Demux3/1
  Demux3/3 -> [TL_DZDX]
  Demux3/1 -> [FL_DZDX]
  Demux3/2 -> [FR_DZDX]
  Demux4/2 -> [FR_DZDY]
  Demux4/4 -> [TR_DZDY]
  Demux4/1 -> [FL_DZDY]
  Demux4/3 -> [TL_DZDY]
  In6/1 -> Demux4/1
  Demux5/3 -> [TL_MU]
  Demux5/4 -> [TR_MU]
  Demux5/2 -> [FR_MU]
  Demux5/1 -> [FL_MU]
  In5/1 -> Demux5/1
  [FL_X] -> front_left/1(xarry)
  [FL_Y] -> front_left/2(yarray)
  [FL_MU] -> front_left/6(muarray)
  [FL_DZDY] -> front_left/5(dzdyarray)
  [FL_DZDX] -> front_left/4(dzdxarray)
  [FL_Z] -> front_left/3(zarray)
  [FR_X] -> front_right/1(xarry)
  [FR_Y] -> front_right/2(yarray)
  [FR_Z] -> front_right/3(zarray)
  [FR_DZDX] -> front_right/4(dzdxarray)
  [FR_DZDY] -> front_right/5(dzdyarray)
  [FR_MU] -> front_right/6(muarray)
  [TL_X] -> tail_left/1(xarry)
  [TL_Y] -> tail_left/2(yarray)
  [TL_Z] -> tail_left/3(zarray)
  [TL_DZDX] -> tail_left/4(dzdxarray)
  [TL_DZDY] -> tail_left/5(dzdyarray)
  [TL_MU] -> tail_left/6(muarray)
  [TR_X] -> tail_right/1(xarry)
  [TR_Y] -> tail_right/2(yarray)
  [TR_Z] -> tail_right/3(zarray)
  [TR_DZDX] -> tail_right/4(dzdxarray)
  [TR_DZDY] -> tail_right/5(dzdyarray)
  [TR_MU] -> tail_right/6(muarray)
  front_left/1(out) -> front_right1/1(fl)
  front_right/1(out) -> front_right1/2(fr)
  front_right1/1(z) -> AddHeight/2(roadZ)
  front_right1/2(dzdx) -> dzdx/1
  front_right1/3(dzdy) -> dzdy/1
  front_right1/4(mu) -> mu/1
  tail_left/1(out) -> front_right1/3(tl)
  tail_right/1(out) -> front_right1/4(tr)
  P1/1 -> [P1]
  Demux6/1 -> front_left/7(x)
  Demux6/2 -> front_left/8(y)
  P2/1 -> [P2]
  Demux7/1 -> front_right/7(x)
  Demux7/2 -> front_right/8(y)
  Demux8/1 -> tail_left/7(x)
  Demux8/2 -> tail_left/8(y)
  P3/1 -> [P3]
  Demux9/1 -> tail_right/7(x)
  Demux9/2 -> tail_right/8(y)
  P4/1 -> [P4]

== system ACCSampleSimulink/Veh_1/ComplexVehicleModel/RoadInfo/Subsystem1 ==
  Rx_eo2ctc_coE_Refine : Inport
  Ry_eo2ctc_coE_Refine : Inport  Port=2
  front_right : MATLAB Function  TreatAsAtomicUnit=on
  P1 : Outport  VectorParamsAs1DForOutWhenUnconnected=off
  P2 : Outport  Port=2  VectorParamsAs1DForOutWhenUnconnected=off
  P3 : Outport  Port=3  VectorParamsAs1DForOutWhenUnconnected=off
  P4 : Outport  Port=4  VectorParamsAs1DForOutWhenUnconnected=off
  wires:
  Rx_eo2ctc_coE_Refine/1 -> front_right/1(array1)
  Ry_eo2ctc_coE_Refine/1 -> front_right/2(array2)
  front_right/2(p2) -> P2/1
  front_right/1(p1) -> P1/1
  front_right/3(p3) -> P3/1
  front_right/4(p4) -> P4/1

== system ACCSampleSimulink/Veh_1/VehicleDataBus/GlobalVariableWrite/GlobalVariableSwitch ==
  value : Inport
  time : Inport  Port=2
  originalValue : Inport  Port=3
  originalTime : Inport  Port=4
  GlobalVariable0 : S-Function  FunctionName=BusWriter  Parameters='global.0','time@i,variable@d','0.01','0.0'  SFunctionDeploymentMode=off  EnableBusSupport=off
  Minus : Sum  Inputs=+-
  Switch : Switch  Criteria=u2 ~= 0  Threshold=1  SaturateOnIntegerOverflow=off  InputSameDT=off
  wires:
  Switch/1 -> GlobalVariable0/1
  originalTime/1 -> Switch/3
  time/1 -> Switch/1
  Minus/1 -> Switch/2
  originalValue/1 -> Minus/2
  value/1 -> Minus/1, GlobalVariable0/2

== system ACCSampleSimulink/Veh_1/VehicleDataBus/GlobalVariableWrite/GlobalVariableSwitch1 ==
  value : Inport
  time : Inport  Port=2
  originalValue : Inport  Port=3
  originalTime : Inport  Port=4
  GlobalVariable1 : S-Function  FunctionName=BusWriter  Parameters='global.1','time@i,variable@d','0.01','0.0'  SFunctionDeploymentMode=off  EnableBusSupport=off
  Minus : Sum  Inputs=+-
  Switch : Switch  Criteria=u2 ~= 0  Threshold=1  SaturateOnIntegerOverflow=off  InputSameDT=off
  wires:
  Switch/1 -> GlobalVariable1/1
  originalTime/1 -> Switch/3
  time/1 -> Switch/1
  Minus/1 -> Switch/2
  originalValue/1 -> Minus/2
  value/1 -> Minus/1, GlobalVariable1/2

== system ACCSampleSimulink/Veh_1/VehicleDataBus/GlobalVariableWrite/GlobalVariableSwitch2 ==
  value : Inport
  time : Inport  Port=2
  originalValue : Inport  Port=3
  originalTime : Inport  Port=4
  GlobalVariable2 : S-Function  FunctionName=BusWriter  Parameters='global.2','time@i,variable@d','0.01','0.0'  SFunctionDeploymentMode=off  EnableBusSupport=off
  Minus : Sum  Inputs=+-
  Switch : Switch  Criteria=u2 ~= 0  Threshold=1  SaturateOnIntegerOverflow=off  InputSameDT=off
  wires:
  Switch/1 -> GlobalVariable2/1
  originalTime/1 -> Switch/3
  time/1 -> Switch/1
  Minus/1 -> Switch/2
  originalValue/1 -> Minus/2
  value/1 -> Minus/1, GlobalVariable2/2

== system ACCSampleSimulink/Veh_1/VehicleDataBus/GlobalVariableWrite/GlobalVariableSwitch3 ==
  value : Inport
  time : Inport  Port=2
  originalValue : Inport  Port=3
  originalTime : Inport  Port=4
  GlobalVariable3 : S-Function  FunctionName=BusWriter  Parameters='global.3','time@i,variable@d','0.01','0.0'  SFunctionDeploymentMode=off  EnableBusSupport=off
  Minus : Sum  Inputs=+-
  Switch : Switch  Criteria=u2 ~= 0  Threshold=1  SaturateOnIntegerOverflow=off  InputSameDT=off
  wires:
  Switch/1 -> GlobalVariable3/1
  originalTime/1 -> Switch/3
  time/1 -> Switch/1
  Minus/1 -> Switch/2
  originalValue/1 -> Minus/2
  value/1 -> Minus/1, GlobalVariable3/2

== system ACCSampleSimulink/Veh_1/VehicleDataBus/GlobalVariableWrite/GlobalVariableSwitch4 ==
  value : Inport
  time : Inport  Port=2
  originalValue : Inport  Port=3
  originalTime : Inport  Port=4
  GlobalVariable4 : S-Function  FunctionName=BusWriter  Parameters='global.4','time@i,variable@d','0.01','0.0'  SFunctionDeploymentMode=off  EnableBusSupport=off
  Minus : Sum  Inputs=+-
  Switch : Switch  Criteria=u2 ~= 0  Threshold=1  SaturateOnIntegerOverflow=off  InputSameDT=off
  wires:
  Switch/1 -> GlobalVariable4/1
  originalTime/1 -> Switch/3
  time/1 -> Switch/1
  Minus/1 -> Switch/2
  originalValue/1 -> Minus/2
  value/1 -> Minus/1, GlobalVariable4/2

== system ACCSampleSimulink/Veh_1/VehicleDataBus/GlobalVariableWrite/GlobalVariableSwitch5 ==
  value : Inport
  time : Inport  Port=2
  originalValue : Inport  Port=3
  originalTime : Inport  Port=4
  GlobalVariable5 : S-Function  FunctionName=BusWriter  Parameters='global.5','time@i,variable@d','0.01','0.0'  SFunctionDeploymentMode=off  EnableBusSupport=off
  Minus : Sum  Inputs=+-
  Switch : Switch  Criteria=u2 ~= 0  Threshold=1  SaturateOnIntegerOverflow=off  InputSameDT=off
  wires:
  Switch/1 -> GlobalVariable5/1
  originalTime/1 -> Switch/3
  time/1 -> Switch/1
  Minus/1 -> Switch/2
  originalValue/1 -> Minus/2
  value/1 -> Minus/1, GlobalVariable5/2

== system ACCSampleSimulink/Veh_1/VehicleDataBus/GlobalVariableWrite/GlobalVariableSwitch6 ==
  value : Inport
  time : Inport  Port=2
  originalValue : Inport  Port=3
  originalTime : Inport  Port=4
  GlobalVariable6 : S-Function  FunctionName=BusWriter  Parameters='global.6','time@i,variable@d','0.01','0.0'  SFunctionDeploymentMode=off  EnableBusSupport=off
  Minus : Sum  Inputs=+-
  Switch : Switch  Criteria=u2 ~= 0  Threshold=1  SaturateOnIntegerOverflow=off  InputSameDT=off
  wires:
  Switch/1 -> GlobalVariable6/1
  originalTime/1 -> Switch/3
  time/1 -> Switch/1
  Minus/1 -> Switch/2
  originalValue/1 -> Minus/2
  value/1 -> Minus/1, GlobalVariable6/2

== system ACCSampleSimulink/Veh_1/VehicleDataBus/GlobalVariableWrite/GlobalVariableSwitch7 ==
  value : Inport
  time : Inport  Port=2
  originalValue : Inport  Port=3
  originalTime : Inport  Port=4
  GlobalVariable7 : S-Function  FunctionName=BusWriter  Parameters='global.7','time@i,variable@d','0.01','0.0'  SFunctionDeploymentMode=off  EnableBusSupport=off
  Minus : Sum  Inputs=+-
  Switch : Switch  Criteria=u2 ~= 0  Threshold=1  SaturateOnIntegerOverflow=off  InputSameDT=off
  wires:
  Switch/1 -> GlobalVariable7/1
  originalTime/1 -> Switch/3
  time/1 -> Switch/1
  Minus/1 -> Switch/2
  originalValue/1 -> Minus/2
  value/1 -> Minus/1, GlobalVariable7/2

== system ACCSampleSimulink/Veh_1/VehicleDataBus/GlobalVariableWrite/GlobalVariableSwitch8 ==
  value : Inport
  time : Inport  Port=2
  originalValue : Inport  Port=3
  originalTime : Inport  Port=4
  GlobalVariable8 : S-Function  FunctionName=BusWriter  Parameters='global.8','time@i,variable@d','0.01','0.0'  SFunctionDeploymentMode=off  EnableBusSupport=off
  Minus : Sum  Inputs=+-
  Switch : Switch  Criteria=u2 ~= 0  Threshold=1  SaturateOnIntegerOverflow=off  InputSameDT=off
  wires:
  Switch/1 -> GlobalVariable8/1
  originalTime/1 -> Switch/3
  time/1 -> Switch/1
  Minus/1 -> Switch/2
  originalValue/1 -> Minus/2
  value/1 -> Minus/1, GlobalVariable8/2

== system ACCSampleSimulink/Veh_1/VehicleDataBus/GlobalVariableWrite/GlobalVariableSwitch9 ==
  value : Inport
  time : Inport  Port=2
  originalValue : Inport  Port=3
  originalTime : Inport  Port=4
  GlobalVariable9 : S-Function  FunctionName=BusWriter  Parameters='global.9','time@i,variable@d','0.01','0.0'  SFunctionDeploymentMode=off  EnableBusSupport=off
  Minus : Sum  Inputs=+-
  Switch : Switch  Criteria=u2 ~= 0  Threshold=1  SaturateOnIntegerOverflow=off  InputSameDT=off
  wires:
  Switch/1 -> GlobalVariable9/1
  originalTime/1 -> Switch/3
  time/1 -> Switch/1
  Minus/1 -> Switch/2
  originalValue/1 -> Minus/2
  value/1 -> Minus/1, GlobalVariable9/2

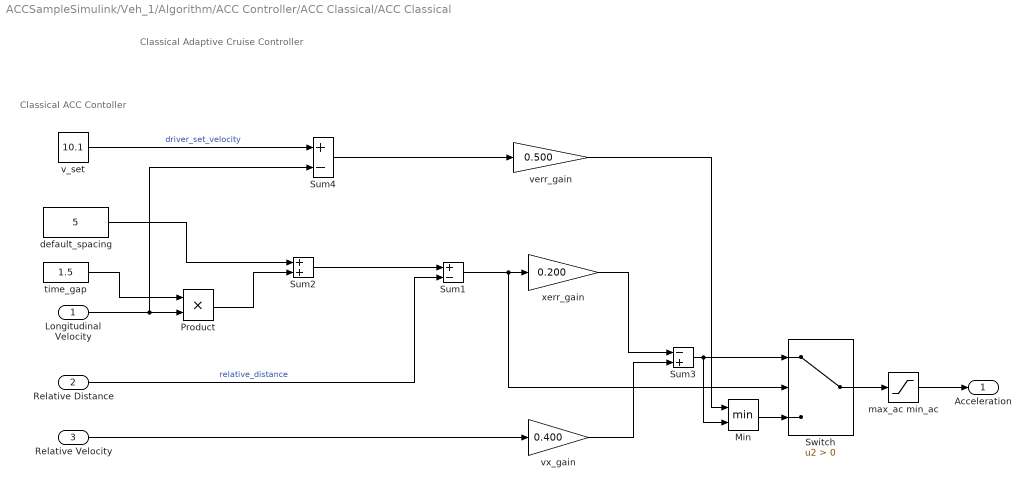
== system ACCSampleSimulink/Veh_1/Algorithm/ACC Controller/ACC Classical/ACC Classical ==
  note: Classical ACC Contoller
  note: Classical Adaptive Cruise Controller
  Longitudinal Velocity : Inport
  Relative Distance : Inport  Port=2
  Relative Velocity : Inport  Port=3
  Min : MinMax  Inputs=2
  Product : Product
  Sum1 : Sum  Inputs=+-
  Sum2 : Sum
  Sum3 : Sum  Inputs=-+
  Sum4 : Sum  Inputs=+-
  Switch : Switch  Criteria=u2 > Threshold  SaturateOnIntegerOverflow=off  InputSameDT=off
  default_spacing : Constant  Value=5
  max_ac min_ac : Saturate  UpperLimit=2  LowerLimit=-3
  time_gap : Constant  Value=1.5
  v_set : Constant  Value=10.1
  verr_gain : Gain  Gain=0.500
  vx_gain : Gain  Gain=0.400
  xerr_gain : Gain  Gain=0.200
  Acceleration : Outport  VectorParamsAs1DForOutWhenUnconnected=off
  wires:
  Longitudinal Velocity/1 -> Product/2, Sum4/2
  default_spacing/1 -> Sum2/1
  xerr_gain/1 -> Sum3/1
  Sum4/1 -> verr_gain/1
  Min/1 -> Switch/3
  vx_gain/1 -> Sum3/2
  Switch/1 -> max_ac min_ac/1
  Relative Velocity/1 -> vx_gain/1
  time_gap/1 -> Product/1
  max_ac min_ac/1 -> Acceleration/1
  Product/1 -> Sum2/2
  v_set/1 -> Sum4/1  "driver_set_velocity"
  Sum3/1 -> Min/2, Switch/1
  Sum1/1 -> Switch/2, xerr_gain/1
  verr_gain/1 -> Min/1
  Relative Distance/1 -> Sum1/2  "relative_distance"
  Sum2/1 -> Sum1/1

== matlab function ACCSampleSimulink/Veh_1/ComplexVehicleModel/RoadInfo/Subsystem/front_right1 ==
  data: z output double; fl input; fr input; tl input; tr input; dzdx output; dzdy output; mu output
function [z,dzdx,dzdy,mu]  = fcn(fl,fr,tl,tr)
    z =  [fl(1),fr(1),tl(1),tr(1)];
    dzdx = [fl(2),fr(2),tl(2),tr(2)];
    dzdy = [fl(3),fr(3),tl(3),tr(3)];
    mu =   [fl(4),fr(4),tl(4),tr(4)];
end

== matlab function ACCSampleSimulink/Veh_1/ComplexVehicleModel/RoadInfo/Subsystem1/front_right ==
  data: p1 output double; array1 input; array2 input; p2 output; p3 output; p4 output
function [p1,p2,p3,p4]  = fcn(array1,array2)
    p1 = [array1(1),array2(1)];
    p2 = [array1(2),array2(2)];
    p3 = [array1(3),array2(3)];
    p4 = [array1(4),array2(4)];
end

== matlab function ACCSampleSimulink/Veh_1/ComplexVehicleModel/RoadInfo/Subsystem/Cal_Height ==
  data: retHeight output double; bumsNum input; x1array input; y1array input; x2array input; y2array input; x3array input; y3array input; x4array input; y4array input; heightarray input; px0 input; py0 input; px1 input; py1 input; px2 input; py2 input; px3 input; py3 input; retValue output
function [retHeight,retValue]   = fcn(bumsNum,x1array,y1array,x2array,y2array,x3array,y3array,x4array,y4array,heightarray,px0,py0,px1,py1,px2,py2,px3,py3)
h0 = 0.0;
h1 = 0.0;
h2 = 0.0;
h3 = 0.0;
value0 = 0;
value1 = 0;
value2 = 0;
value3 = 0;
for index = 1:bumsNum+1
     v = fcn_in_sqar(x1array(index),y1array(index),x2array(index),y2array(index),x3array(index),y3array(index),x4array(index),y4array(index),px0,py0);
     if (v > 0)
         value0 = 1;
         h0 =  heightarray(index);
         break;
     end
end
for index = 1:bumsNum+1
     v = fcn_in_sqar(x1array(index),y1array(index),x2array(index),y2array(index),x3array(index),y3array(index),x4array(index),y4array(index),px1,py1);
     if (v > 0)
         value1 = 1;
         h1 =  heightarray(index);
         break;
     end
end

for index = 1:bumsNum+1
     v = fcn_in_sqar(x1array(index),y1array(index),x2array(index),y2array(index),x3array(index),y3array(index),x4array(index),y4array(index),px2,py2);
     if (v > 0)
         value2 = 1;
         h2 =  heightarray(index);
         break;
     end
end

for index = 1:bumsNum+1
     v = fcn_in_sqar(x1array(index),y1array(index),x2array(index),y2array(index),x3array(index),y3array(index),x4array(index),y4array(index),px3,py3);
     if (v > 0)
         value3 = 1;
         h3 =  heightarray(index);
         break;
     end
end
retHeight = [h0,h1,h2,h3];
retValue = [value0,value1,value2,value3];
end


function ret = fcn_in_sqar(x1,y1,x2,y2,x3,y3,x4,y4,x,y)
    ret = 0;
    a = (x2-x1)*(y-y1)-(y2-y1)*(x-x1);
    b = (x3-x2)*(y-y2)-(y3-y2)*(x-x2);
    c = (x4-x3)*(y-y3)-(y4-y3)*(x-x3);
    d = (x1-x4)*(y-y4)-(y1-y4)*(x-x4);
    if (a>=0&&b>=0&&c>=0&&d>=0)
        ret = 1;
    end
    if (a<=0&&b<=0&&c<=0&&d<=0)
        ret = 1;
    end
end

== matlab function ACCSampleSimulink/Veh_1/ComplexVehicleModel/RoadInfo/Subsystem/AddHeight ==
  data: z output double; height input; roadZ input
function z  = fcn(height,roadZ)
    z =  [roadZ(1)+height(1),roadZ(2)+height(2),roadZ(3)+height(3),roadZ(4)+height(4)];
end

== matlab function ACCSampleSimulink/Veh_1/Algorithm/ControlSignalFilter/MATLAB Function ==
  data: driver input; valid output; algoThrottle input; algoBrake input; algoSteer input; algoMode input; algoGear input; throttle output; brake output; steer output; mode output; gear output
function [valid,throttle,brake,steer,mode,gear] = fcn(driver,algoThrottle,algoBrake,algoSteer,algoMode,algoGear)
valid = driver(1) + algoThrottle(2) + algoBrake(2) + algoSteer(2) + algoMode(2) + algoGear(2);
if valid > 0
    valid = 1;
end

throttle = fcnValidData(driver(2),algoThrottle(3),algoThrottle(2));
brake = fcnValidData(driver(3),algoBrake(3),algoBrake(2));
steer = fcnValidData(driver(4),algoSteer(3),algoSteer(2));
mode = fcnValidData(driver(5),algoMode(3),algoMode(2));
gear = fcnValidData(driver(6),algoGear(3),algoGear(2));

end

function out = fcnValidData(data1,data2,valid)
    if valid > 0.5
        out = data2;
    else
        out = data1;
    end
end
